simulink model "Model5"  (R2020a)
settings: Solver=VariableStepAuto  StartTime=0.0  StopTime=1.302083333333333e-14  RelTol=1e-3
undefined symbols (not defined in the file or in its folder): doppler, pskmod
libraries: commutil2 x4, commdigbbndpm3 x3, commchan3 x2, commsink2 x2, commrandsrc3 x1, commrflib2 x1
settings Model: Creator=esha_  LastModifiedBy=esha_

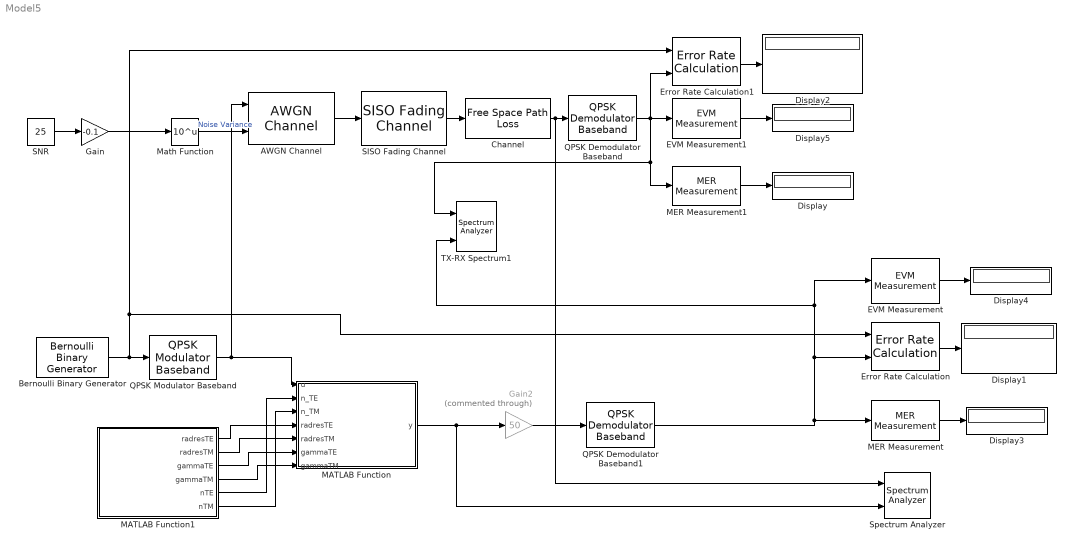
== system Model5 ==
  AWGN Channel : commchan3/AWGN Channel  InputProcessing=Columns as channels (frame based)  seed=67  noiseMode=Variance from port  EbNodB=1  EsNodB=10  SNRdB=10  bitsPerSym=1  Ps=0.001  Tsym=0.000000065  variance=1
  Bernoulli Binary Generator : commrandsrc3/Bernoulli Binary Generator  ProbabilityOfZero=0.5  SeedSource=Parameter  Seed=61  SampleTime=1.302083333333333e-07  SamplesPerFrame=10000  OutputDataType=double  SimulateUsing=Code generation
  Channel : commrflib2/Free Space Path Loss  mode=Decibels  dB=70  d=0.100  fc=1920
      settings: SourceProductBaseCode=CM
  Display{,1..5} (6 alike) : Display
  EVM Measurement : commutil2/EVM Measurement  Normalization=Average reference signal power  AverageConstellationPower=1  PeakConstellationPower=1  ReferenceSignalSource=Estimated from reference constellation  ReferenceConstellation=pskmod((0:1),2,0)  MeasurementIntervalSource=Input length  MeasurementInterval=100  AveragingDimensions=1  MaximumEVMOutputPort=off  XPercentileEVMOutputPort=off  XPercentileValue=95  SymbolCountOutputPort=on  SimulateUsing=Interpreted execution
      settings: SourceProductBaseCode=CM
  EVM Measurement1 : commutil2/EVM Measurement  Normalization=Average reference signal power  AverageConstellationPower=1  PeakConstellationPower=1  ReferenceSignalSource=Estimated from reference constellation  ReferenceConstellation=pskmod((0:1),2,0)  MeasurementIntervalSource=Input length  MeasurementInterval=100  AveragingDimensions=1  MaximumEVMOutputPort=off  XPercentileEVMOutputPort=off  XPercentileValue=95  SymbolCountOutputPort=on  SimulateUsing=Interpreted execution
      settings: SourceProductBaseCode=CM
  Error Rate Calculation : commsink2/Error Rate Calculation  N=0  st_delay=0  cp_mode=Entire frame  subframe=[]  PMode=Port  WsName=ErrorVec  RsMode2=off  stop=off  numErr=100  maxBits=1e6
  Error Rate Calculation1 : commsink2/Error Rate Calculation  N=0  st_delay=0  cp_mode=Entire frame  subframe=[]  PMode=Port  WsName=ErrorVec  RsMode2=off  stop=off  numErr=100  maxBits=1e6
  Gain : Gain  Gain=-0.1
  Gain2 : Gain  Commented=through  Gain=50
  MATLAB Function : MATLAB Function  TreatAsAtomicUnit=on
  MATLAB Function1 : MATLAB Function  TreatAsAtomicUnit=on
  MER Measurement : commutil2/MER Measurement  ReferenceSignalSource=Estimated from reference constellation  ReferenceConstellation=pskmod((0:1),2,0)  MeasurementIntervalSource=Input length  MeasurementInterval=100  AveragingDimensions=1  MinimumMEROutputPort=off  XPercentileMEROutputPort=off  XPercentileValue=95  SymbolCountOutputPort=off  SimulateUsing=Interpreted execution
      settings: SourceProductBaseCode=CM
  MER Measurement1 : commutil2/MER Measurement  ReferenceSignalSource=Estimated from reference constellation  ReferenceConstellation=pskmod((0:1),2,0)  MeasurementIntervalSource=Input length  MeasurementInterval=100  AveragingDimensions=1  MinimumMEROutputPort=off  XPercentileMEROutputPort=off  XPercentileValue=95  SymbolCountOutputPort=off  SimulateUsing=Interpreted execution
      settings: SourceProductBaseCode=CM
  Math Function : Math  Operator=10^u  SignedPower=on  SaturateOnIntegerOverflow=on
  QPSK Demodulator Baseband : commdigbbndpm3/QPSK Demodulator Baseband  OutType=Bit  DecType=Hard decision  VarSource=Dialog  Variance=1  Dec=Binary  Ph=pi/4  outDtype1=Inherit via internal rule  outDtype2=Inherit via internal rule  derotateFactorWordLen=16  derotateFactorDataTypeStr=Inherit: Same word length as input  derotateFactorLastDataTypeStr=Inherit: Same word length as input
  QPSK Demodulator Baseband1 : commdigbbndpm3/QPSK Demodulator Baseband  OutType=Bit  DecType=Hard decision  VarSource=Dialog  Variance=1  Dec=Binary  Ph=pi/4  outDtype1=Inherit via internal rule  outDtype2=Inherit via internal rule  derotateFactorWordLen=16  derotateFactorDataTypeStr=Inherit: Same word length as input  derotateFactorLastDataTypeStr=Inherit: Same word length as input
  QPSK Modulator Baseband : commdigbbndpm3/QPSK Modulator Baseband  InType=Bit  Enc=Binary  Ph=pi/4  outDtype=double  outWordLen=16  outUDDataType=sfix(16)  outFracLenMode=Best precision  outFracLen=15  outDataTypeStr=double  outLastDataTypeStr=double
  SISO Fading Channel : commchan3/SISO Fading Channel  InheritSampleRate=on  SampleRate=1  PathDelays="[0\t2.00E-07\t4.00E-07\t6.00E-07\t8.00E-07\t1.00E-06\t1.20E-06\t1.40E-06\t1.60E-06\t1.80E-06\t2.00E-06\t2.20E-06\t2.40E-06\t2.60E-06\t2.80E-06\t3.00E-06\t3.20E-06\t3.40E-06\t3.60E-06\t3.80E-06\t4.00E-06\t4.20E-06\t4.40E-06\t4.60E-06\t4.80E-06\t5.00E-06\t5.20E-06\t5.40E-06\t5.60E-06\t5.80E-06\t6.00E-06\t6.20E-06\t6.40E-06\t6.60E-06\t6.80E-06\t7.00E-06\t7.20E-06\t7.40E-06\t7.60E-06\t7.80E-06\t8.00E-06\t8.20E-06\t8.40E-06\t8.60E-06\t8.80E-06\t9.00E-06\t9.20E-06\t9.40E-06\t9.60E-06\t9.80E-06\t1.00E-05\t1.02E-05\t1.04E-05\t1.06E-05\t1.08E-05\t1.10E-05\t1.12E-05\t1.14E-05\t1.16E-05\t1.18E-05\t1.20E-05\t1.22E-05\t1.24E-05\t1.26E-05\t1.28E-05\t1.30E-05\t1.32E-05\t1.34E-05\t1.36E-05\t1.38E-05\t1.40E-05\t1.42E-05\t1.44E-05\t1.46E-05\t1.48E-05\t1.50E-05\t1.52E-05\t1.54E-05\t1.56E-05\t1.58E-05\t1.60E-05\t1.62E-05\t1.64E-05\t1.66E-05\t1.68E-05\t1.70E-05\t1.72E-05\t1.74E-05\t1.76E-05\t1.78E-05\t1.80E-05\t1.82E-05\t1.84E-05\t1.86E-05\t1.88E-05\t1.90E-05\t1.92E-05\t1.94E-05\t1.96E-05\t1.98E-05\t2.00E-05\t2.02E-05\t2.04E-05\t2.06E-05\t2.08E-05\t2.10E-05\t2.12E-05\t2.14E-05\t2.16E-05\t2.18E-05\t2.20E-05\t2.22E-05\t2.24E-05\t2.26E-05\t2.28E-05\t2.30E-05\t2.32E-05\t2.34E-05\t2.36E-05\t2.38E-05\t2.40E-05\t2.42E-05\t2.44E-05\t2.46E-05\t2.48E-05\t2.50E-05\t2.52E-05\t2.54E-05\t2.56E-05\t2.58E-05\t2.60E-05\t2.62E-05\t2.64E-05\t2.66E-05\t2.68E-05\t2.70E-05\t2.72E-05\t2.74E-05\t2.76E-05\t2.78E-05\t2.80E-05\t2.82E-05\t2.84E-05\t2.86E-05\t2.88E-05\t2.90E-05\t2.92E-05\t2.94E-05\t2.96E-05\t2.98E-05\t3.00E-05\t3.02E-05\t3.04E-05\t3.06E-05\t3.08E-05\t3.10E-05\t3.12E-05\t3.14E-05\t3.16E-05\t3.18E-05\t3.20E-05\t3.22E-05\t3.24E-05\t3.26E-05\t3.28E-05\t3.30E-05\t3.32E-05\t3.34E-05\t3.36E-05\t3.38E-05\t3.40E-05\t3.42E-05\t3.44E-05\t3.46E-05\t3.48E-05\t3.50E-05\t3.52E-05\t3.54E-05\t3.56E-05\t3.58E-05\t3.60E-05\t3.62E-05\t3.64E-05\t3.66E-05\t3.68E-05\t3.70E-05\t3.72E-05\t3.74E-05\t3.76E-05\t3.78E-05\t3.80E-05\t3.82E-05\t3.84E-05\t3.86E-05\t3.88E-05\t3.90E-05\t3.92E-05\t3.94E-05\t3.96E-05\t3.98E-05]"  AveragePathGains="[0\t-1\t-2\t-3\t-4\t-5\t-6\t-7\t-8\t-9\t-10\t-11\t-12\t-13\t-14\t-15\t-16\t-17\t-18\t-19\t-20\t-21\t-22\t-23\t-24\t-25\t-26\t-27\t-28\t-29\t-30\t-31\t-32\t-33\t-34\t-35\t-36\t-37\t-38\t-39\t-40\t-41\t-42\t-43\t-44\t-45\t-46\t-47\t-48\t-49\t-50\t-51\t-52\t-53\t-54\t-55\t-56\t-57\t-58\t-59\t-60\t-61\t-62\t-63\t-64\t-65\t-66\t-67\t-68\t-69\t-70\t-71\t-72\t-73\t-74\t-75\t-76\t-77\t-78\t-79\t-80\t-81\t-82\t-83\t-84\t-85\t-86\t-87\t-88\t-89\t-90\t-91\t-92\t-93\t-94\t-95\t-96\t-97\t-98\t-99\t-100\t-101\t-102\t-103\t-104\t-105\t-106\t-107\t-108\t-109\t-110\t-111\t-112\t-113\t-114\t-115\t-116\t-117\t-118\t-119\t-120\t-121\t-122\t-123\t-124\t-125\t-126\t-127\t-128\t-129\t-130\t-131\t-132\t-133\t-134\t-135\t-136\t-137\t-138\t-139\t-140\t-141\t-142\t-143\t-144\t-145\t-146\t-147\t-148\t-149\t-150\t-151\t-152\t-153\t-154\t-155\t-156\t-157\t-158\t-159\t-160\t-161\t-162\t-163\t-164\t-165\t-166\t-167\t-168\t-169\t-170\t-171\t-172\t-173\t-174\t-175\t-176\t-177\t-178\t-179\t-180\t-181\t-182\t-183\t-184\t-185\t-186\t-187\t-188\t-189\t-190\t-191\t-192\t-193\t-194\t-195\t-196\t-197\t-198\t-199]"  NormalizePathGains=on  FadingDistribution=Rayleigh  KFactor=3  DirectPathDopplerShift=0  DirectPathInitialPhase=0  MaximumDopplerShift=0.001  DopplerSpectrum=doppler('Jakes')  RandomStream=mt19937ar with seed  Seed=61  PathGainsOutputPort=off  ChannelFilterDelayOutputPort=off  SimulateUsing=Interpreted execution  Visualization=Frequency response  PathsForDopplerDisplay=1  SamplesToDisplay=100%
  SNR : Constant  Value=25
  Spectrum Analyzer : SpectrumAnalyzer  NumInputPorts=2
  TX-RX Spectrum1 : SpectrumAnalyzer  NumInputPorts=2
  wires:
  SNR/1 -> Gain/1
  EVM Measurement/1 -> Display4/1
  EVM Measurement1/1 -> Display5/1
  AWGN Channel/1 -> SISO Fading Channel/1
  MER Measurement/1 -> Display3/1
  MATLAB Function1/5(nTE) -> MATLAB Function/2(n_TE)
  MATLAB Function1/6(nTM) -> MATLAB Function/3(n_TM)
  MATLAB Function1/1(radresTE) -> MATLAB Function/4(radresTE)
  QPSK Demodulator Baseband/1 -> EVM Measurement1/1, Error Rate Calculation1/2, TX-RX Spectrum1/1, MER Measurement1/1
  MER Measurement1/1 -> Display/1
  SISO Fading Channel/1 -> Channel/1
  Bernoulli Binary Generator/1 -> QPSK Modulator Baseband/1, Error Rate Calculation1/1, Error Rate Calculation/1
  Gain/1 -> Math Function/1
  MATLAB Function1/3(gammaTE) -> MATLAB Function/6(gammaTE)
  Channel/1 -> QPSK Demodulator Baseband/1, Spectrum Analyzer/1
  Math Function/1 -> AWGN Channel/2  "Noise Variance"
  MATLAB Function1/4(gammaTM) -> MATLAB Function/7(gammaTM)
  Error Rate Calculation1/1 -> Display2/1
  Error Rate Calculation/1 -> Display1/1
  MATLAB Function1/2(radresTM) -> MATLAB Function/5(radresTM)
  QPSK Modulator Baseband/1 -> MATLAB Function/1(u), AWGN Channel/1
  Gain2/1 -> QPSK Demodulator Baseband1/1
  MATLAB Function/1(y) -> Gain2/1, Spectrum Analyzer/2
  QPSK Demodulator Baseband1/1 -> MER Measurement/1, TX-RX Spectrum1/2, EVM Measurement/1, Error Rate Calculation/2

== matlab function Model5/MATLAB Function1 ==
  data: radresTE output; radresTM output; gammaTE output; gammaTM output; nTE output; nTM output
function [radresTE, radresTM, gammaTE, gammaTM, nTE, nTM] = fcn()
nTE1 = load('nTE.mat');
nTE = nTE1.n_TE;
nTM1 = load('nTM.mat');
nTM = nTM1.n_TM;
radresTE1 = load('radresTE.mat');
radresTE = radresTE1.radresTES;
radresTM1 = load('radresTM.mat');
radresTM = radresTM1.radresTMS;
gammaTE1 = load('gammaTE.mat');
gammaTE = gammaTE1.gammaTES;
gammaTM1 = load('gammaTM.mat');
gammaTM = gammaTM1.gammaTMS;
end

== matlab function Model5/MATLAB Function ==
  data: y output; u input; n_TE input; n_TM input; radresTE input; radresTM input; gammaTE input; gammaTM input
function y = fcn(u,n_TE, n_TM, radresTE, radresTM, gammaTE, gammaTM)
freq = 59E9:4E6:60E9; 
% n_TE = 0;
% n_TM = 17;
Zo=50;
WGlen = 5;

radreacTE = imag(hilbert(radresTE));
radreacTM = imag(hilbert(radresTM));
antresTE = zeros(1,length(freq));
antresTM = zeros(1,length(freq));
antreacTE = zeros(1,length(freq));
antreacTM = zeros(1,length(freq));
antimpTE = zeros(1,length(freq)) + 1i*zeros(1,length(freq));
antimpTM = zeros(1,length(freq)) + 1i*zeros(1,length(freq));
TEmodeimp = zeros(length(freq), length(n_TE)) + 1i*zeros(length(freq), length(n_TE));
TMmodeimp = zeros(length(freq), length(n_TM)) + 1i*zeros(length(freq), length(n_TM));
channel = zeros(1,length(freq)) + 1i*zeros(1,length(freq));
for fi=1:length(freq)
    antresTE(fi) = sum(radresTE(fi,:));
    antresTM(fi) = sum(radresTM(fi,:));
    antreacTE(fi) = sum(radreacTE(fi,:));
    antreacTM(fi) = sum(radreacTM(fi,:));
    antimpTE(fi) = antresTE(fi) +1i*antreacTE(fi);
    antimpTM(fi) = antresTM(fi) +1i*antreacTM(fi);
    for n = 1:length(n_TE)
        TEmodeimp(fi,n)=radresTE(fi,n)+1i*radreacTE(fi,n);
    end
    for n = 1:length(n_TM)
        TMmodeimp(fi,n)=radresTM(fi,n)+1i*radreacTM(fi,n);
    end    
end
for fi=1:length(freq)
    TsTE = diag(exp(-1*gammaTE(fi,:)*WGlen));
    chTEmode = TEmodeimp(fi,:)*TsTE;
    TsTM = diag(exp(-1*gammaTM(fi,:)*WGlen));
    chTMmode = TMmodeimp(fi,:)*TsTM;
%     channel(fi) = ((2*Zo)/(abs(Zo + antimpTM(fi))^2))*...
%         (sum(chTMmode));
    channel(fi) = ((2*Zo)/(abs(antimpTM(fi) + Zo + antimpTE(fi))^2))*...
        (sum(chTEmode)+sum(chTMmode));
end
 %uu = u';
 cchanel = ((abs(channel)).^2);
 y = zeros(length(u),1);
 for ui = 1:length(u)
     y(ui) = sum(u(ui)*cchanel);
 end
%y = uu.*(cchanel);
% y = conv(u,(abs(channel)).^2,'same');
%y = channel;
